simulink model "sim"  (R2024a)
settings: Solver=VariableStepAuto  StartTime=0.0  StopTime=500  RelTol=1e-3
undefined symbols (not defined in the file): den_cmvk, den_proces, Kr_cmvk, num_cmvk, num_proces
settings Model: Creator=grabo  LastModifiedBy=grabo

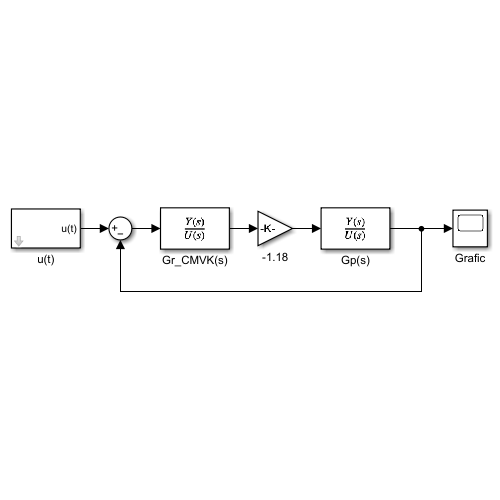
[thumbnail: Simulink's stored preview of the top-level diagram]
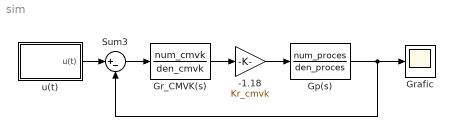
== system sim ==
  -1.18 : Gain  Gain=Kr_cmvk
  Gp(s) : TransferFcn  Numerator=num_proces  Denominator=den_proces
  Gr_CMVK(s) : TransferFcn  Numerator=num_cmvk  Denominator=den_cmvk
  Grafic : Scope
  Sum3 : Sum  Inputs=|+-
  u(t) : Subsystem  mask{With_u=1, Gref=80}
      mask prompts: With_u "With_u ="; Gref "Gref ="
  wires:
  Gp(s)/1 -> Grafic/1, Sum3/2
  Sum3/1 -> Gr_CMVK(s)/1
  u(t)/1(u(t)) -> Sum3/1
  Gr_CMVK(s)/1 -> -1.18/1
  -1.18/1 -> Gp(s)/1

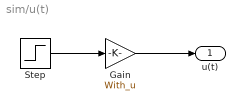
== system sim/u(t) ==
  Gain : Gain  Gain=With_u
  Step : Step  Time=0  After=Gref  SampleTime=0
  u(t) : Outport
  wires:
  Step/1 -> Gain/1
  Gain/1 -> u(t)/1
